simulink model "GammaandTorqueMover"  (R2022b)
settings: Solver=FixedStepAuto  StartTime=0.0  StopTime=10  FixedStep=0.01  RelTol=1e-3
undefined symbols (not defined in the file or in its folder): Kd, Ki, Kp
libraries: mpclib x6, slpidlib x6, simulink x1
(part 2 of 4)

== system GammaandTorqueMover/Tube MPC/MLPM Plant1 ==
  PID Control effort : Inport
  position : Inport  Port=2
  Gamma : Subsystem
  Gravity : Constant  Value=[0;0;-647.2369;0;0;0]
  MATLAB Function : MATLAB Function  TreatAsAtomicUnit=on
  PINV : Subsystem
  Sum1 : Sum  Inputs=++|
  PID Net Wrench : Outport
  PID states : Outport  Port=2
  PID Position and Orientation : Outport  Port=3
  wires:
  Sum1/1 -> MATLAB Function/1(u), PID Net Wrench/1  "PID Net Wrench"
  Gravity/1 -> Sum1/1
  MATLAB Function/2(y) -> PID Position and Orientation/1  "PID Position and Orientation"
  PID Control effort/1 -> PINV/1(input)
  PINV/1(Current) -> Gamma/1(input)  "PID Currents"
  position/1 -> PINV/2(position), Gamma/2(position), MATLAB Function/2(x)
  Gamma/1(net_wrench) -> Sum1/2  "PID Net Wrench"
  MATLAB Function/1(xdot) -> PID states/1  "PID states"

== system GammaandTorqueMover/Tube MPC/Subsystem ==
  Open Loop effort : Inport
  position : Inport  Port=2
  Band-Limited White Noise : simulink/Sources/Band-Limited White Noise  Cov=[0.1]  Ts=0.1  seed=[23341]
  Gamma : Subsystem
  Integrator : Integrator  InitialCondition=[0;0;0;0;0;0;0;0;0;0;0;0]  LimitOutput=on  UpperSaturationLimit=5  LowerSaturationLimit=-5
  MATLAB Function : MATLAB Function  TreatAsAtomicUnit=on
  PINV : Subsystem
  Open Loop Net Wrench : Outport
  Open Loop states : Outport  Port=2
  Open Loop Position and Orientation : Outport  Port=3
  wires:
  Integrator/1 -> Open Loop states/1  "Open Loop states"
  Gamma/1(net_wrench) -> Open Loop Net Wrench/1, MATLAB Function/1(u)  "Open Loop Wrench"
  PINV/1(Current) -> Gamma/1(input)  "Open Loop Currents"
  Open Loop effort/1 -> PINV/1(input)
  MATLAB Function/2(y) -> Open Loop Position and Orientation/1  "Open Loop Position and Orientation"
  position/1 -> MATLAB Function/2(x), Gamma/2(position), PINV/2(position)
  MATLAB Function/1(xdot) -> Integrator/1  "Open Loop states"

== system GammaandTorqueMover/Disturbance added/Linear MPC plus D/MLPM Plant1 ==
  PID Control effort : Inport
  position : Inport  Port=2
  Gamma : Subsystem
  Gravity : Constant  Value=[0;0;-647.2369;0;0;0]
  MATLAB Function : MATLAB Function  TreatAsAtomicUnit=on
  PINV : Subsystem
  Sum1 : Sum  Inputs=++|
  PID Net Wrench : Outport
  PID states : Outport  Port=2
  PID Position and Orientation : Outport  Port=3
  wires:
  Sum1/1 -> MATLAB Function/1(u), PID Net Wrench/1  "PID Net Wrench"
  Gravity/1 -> Sum1/1
  MATLAB Function/2(y) -> PID Position and Orientation/1  "PID Position and Orientation"
  PID Control effort/1 -> PINV/1(input)
  PINV/1(Current) -> Gamma/1(input)  "PID Currents"
  position/1 -> PINV/2(position), Gamma/2(position), MATLAB Function/2(x)
  Gamma/1(net_wrench) -> Sum1/2  "PID Net Wrench"
  MATLAB Function/1(xdot) -> PID states/1  "PID states"

== system GammaandTorqueMover/Disturbance added/Linear MPC plus D/Subsystem ==
  Open Loop effort : Inport
  position : Inport  Port=2
  Gamma : Subsystem
  Integrator : Integrator  InitialCondition=[0;0;0;0;0;0;0;0;0;0;0;0]  LimitOutput=on  UpperSaturationLimit=5  LowerSaturationLimit=-5
  MATLAB Function : MATLAB Function  TreatAsAtomicUnit=on
  Mux2 : Mux  Inputs=6
  PINV : Subsystem
  Step : Step  Time=3  After=1000  SampleTime=0
  Sum : Sum  Inputs=++|
  Open Loop Net Wrench : Outport
  Open Loop states : Outport  Port=2
  Open Loop Position and Orientation : Outport  Port=3
  wires:
  MATLAB Function/1(xdot) -> Integrator/1  "Open Loop states"
  position/1 -> PINV/2(position), Gamma/2(position), MATLAB Function/2(x)
  MATLAB Function/2(y) -> Open Loop Position and Orientation/1  "Open Loop Position and Orientation"
  Open Loop effort/1 -> PINV/1(input)
  PINV/1(Current) -> Gamma/1(input)  "Open Loop Currents"
  Gamma/1(net_wrench) -> Sum/2, Open Loop Net Wrench/1  "Open Loop Wrench"
  Integrator/1 -> Open Loop states/1  "Open Loop states"
  Step/1 -> Mux2/4, Mux2/5, Mux2/6, Mux2/3, Mux2/2, Mux2/1
  Mux2/1 -> Sum/1  "Open loop Disturbance"
  Sum/1 -> MATLAB Function/1(u)

== system GammaandTorqueMover/Disturbance added/PID plus D/MLPM Plant1 ==
  PID Control effort : Inport
  position : Inport  Port=2
  Gamma : Subsystem
  Gravity : Constant  Value=[0;0;-647.2369;0;0;0]
  MATLAB Function : MATLAB Function  TreatAsAtomicUnit=on
  PINV : Subsystem
  Sum1 : Sum  Inputs=++|
  PID Net Wrench : Outport
  PID states : Outport  Port=2
  PID Position and Orientation : Outport  Port=3
  wires:
  MATLAB Function/1(xdot) -> PID states/1  "PID states"
  Gamma/1(net_wrench) -> Sum1/2  "PID Net Wrench"
  position/1 -> MATLAB Function/2(x), Gamma/2(position), PINV/2(position)
  PINV/1(Current) -> Gamma/1(input)  "PID Currents"
  PID Control effort/1 -> PINV/1(input)
  MATLAB Function/2(y) -> PID Position and Orientation/1  "PID Position and Orientation"
  Gravity/1 -> Sum1/1
  Sum1/1 -> PID Net Wrench/1, MATLAB Function/1(u)  "PID Net Wrench"

== system GammaandTorqueMover/Disturbance added/PID plus D/Subsystem ==
  Open Loop effort : Inport
  position : Inport  Port=2
  Gamma : Subsystem
  Integrator : Integrator  InitialCondition=[0;0;0;0;0;0;0;0;0;0;0;0]  LimitOutput=on  UpperSaturationLimit=5  LowerSaturationLimit=-5
  MATLAB Function : MATLAB Function  TreatAsAtomicUnit=on
  Mux2 : Mux  Inputs=6
  PINV : Subsystem
  Step : Step  Time=3  After=1000  SampleTime=0
  Sum : Sum  Inputs=++|
  Open Loop Net Wrench : Outport
  Open Loop states : Outport  Port=2
  Open Loop Position and Orientation : Outport  Port=3
  wires:
  MATLAB Function/1(xdot) -> Integrator/1  "Open Loop states"
  position/1 -> PINV/2(position), Gamma/2(position), MATLAB Function/2(x)
  MATLAB Function/2(y) -> Open Loop Position and Orientation/1  "Open Loop Position and Orientation"
  Open Loop effort/1 -> PINV/1(input)
  PINV/1(Current) -> Gamma/1(input)  "Open Loop Currents"
  Gamma/1(net_wrench) -> Sum/2, Open Loop Net Wrench/1  "Open Loop Wrench"
  Integrator/1 -> Open Loop states/1  "Open Loop states"
  Step/1 -> Mux2/4, Mux2/5, Mux2/6, Mux2/3, Mux2/2, Mux2/1
  Mux2/1 -> Sum/1  "Open loop Disturbance"
  Sum/1 -> MATLAB Function/1(u)

== system GammaandTorqueMover/Disturbance added/Tube MPC plus D/MLPM Plant1 ==
  PID Control effort : Inport
  position : Inport  Port=2
  Gamma : Subsystem
  Gravity : Constant  Value=[0;0;-647.2369;0;0;0]
  MATLAB Function : MATLAB Function  TreatAsAtomicUnit=on
  PINV : Subsystem
  Sum1 : Sum  Inputs=++|
  PID Net Wrench : Outport
  PID states : Outport  Port=2
  PID Position and Orientation : Outport  Port=3
  wires:
  MATLAB Function/1(xdot) -> PID states/1  "PID states"
  Gamma/1(net_wrench) -> Sum1/2  "PID Net Wrench"
  position/1 -> MATLAB Function/2(x), Gamma/2(position), PINV/2(position)
  PINV/1(Current) -> Gamma/1(input)  "PID Currents"
  PID Control effort/1 -> PINV/1(input)
  MATLAB Function/2(y) -> PID Position and Orientation/1  "PID Position and Orientation"
  Gravity/1 -> Sum1/1
  Sum1/1 -> PID Net Wrench/1, MATLAB Function/1(u)  "PID Net Wrench"

== system GammaandTorqueMover/Disturbance added/Tube MPC plus D/Subsystem ==
  Open Loop effort : Inport
  position : Inport  Port=2
  Gamma : Subsystem
  Integrator : Integrator  InitialCondition=[0;0;0;0;0;0;0;0;0;0;0;0]  LimitOutput=on  UpperSaturationLimit=5  LowerSaturationLimit=-5
  MATLAB Function : MATLAB Function  TreatAsAtomicUnit=on
  Mux2 : Mux  Inputs=6
  PINV : Subsystem
  Step : Step  Time=3  After=1000  SampleTime=0
  Sum : Sum  Inputs=++|
  Open Loop Net Wrench : Outport
  Open Loop states : Outport  Port=2
  Open Loop Position and Orientation : Outport  Port=3
  wires:
  MATLAB Function/1(xdot) -> Integrator/1  "Open Loop states"
  position/1 -> PINV/2(position), Gamma/2(position), MATLAB Function/2(x)
  MATLAB Function/2(y) -> Open Loop Position and Orientation/1  "Open Loop Position and Orientation"
  Open Loop effort/1 -> PINV/1(input)
  PINV/1(Current) -> Gamma/1(input)  "Open Loop Currents"
  Gamma/1(net_wrench) -> Sum/2, Open Loop Net Wrench/1  "Open Loop Wrench"
  Integrator/1 -> Open Loop states/1  "Open Loop states"
  Step/1 -> Mux2/4, Mux2/5, Mux2/6, Mux2/3, Mux2/2, Mux2/1
  Mux2/1 -> Sum/1  "Open loop Disturbance"
  Sum/1 -> MATLAB Function/1(u)

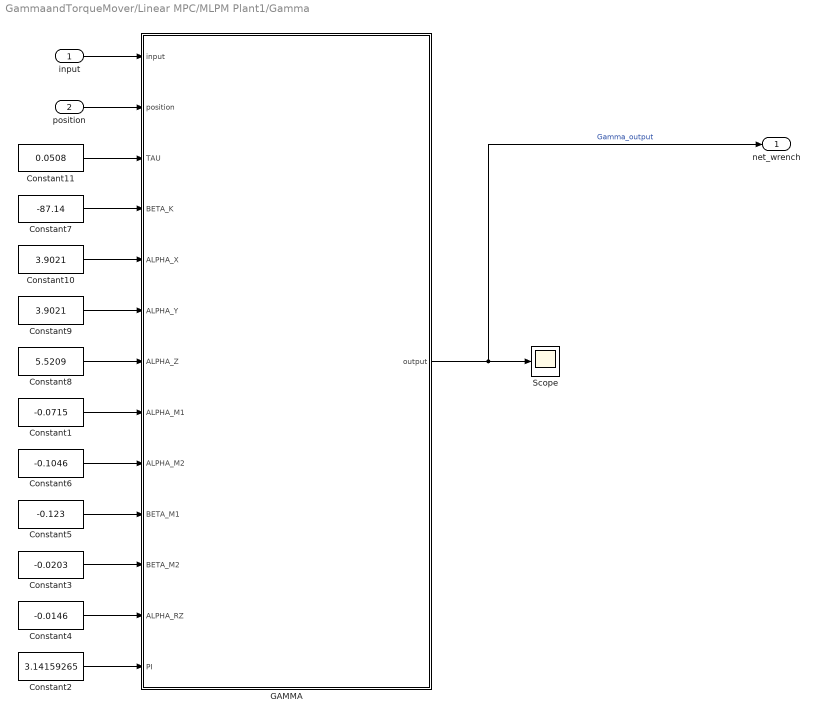
== system GammaandTorqueMover/Linear MPC/MLPM Plant1/Gamma ==
  input : Inport
  position : Inport  Port=2
  Constant1 : Constant  Value=-0.0715
  Constant10 : Constant  Value=3.9021
  Constant11 : Constant  Value=0.0508
  Constant2 : Constant  Value=3.14159265
  Constant3 : Constant  Value=-0.0203
  Constant4 : Constant  Value=-0.0146
  Constant5 : Constant  Value=-0.123
  Constant6 : Constant  Value=-0.1046
  Constant7 : Constant  Value=-87.14
  Constant8 : Constant  Value=5.5209
  Constant9 : Constant  Value=3.9021
  GAMMA : MATLAB Function  TreatAsAtomicUnit=on
  Scope : Scope
  net_wrench : Outport
  wires:
  GAMMA/1(output) -> Scope/1, net_wrench/1  "Gamma_output"
  Constant4/1 -> GAMMA/12(ALPHA_RZ)
  Constant3/1 -> GAMMA/11(BETA_M2)
  Constant5/1 -> GAMMA/10(BETA_M1)
  Constant6/1 -> GAMMA/9(ALPHA_M2)
  Constant1/1 -> GAMMA/8(ALPHA_M1)
  Constant8/1 -> GAMMA/7(ALPHA_Z)
  Constant9/1 -> GAMMA/6(ALPHA_Y)
  Constant10/1 -> GAMMA/5(ALPHA_X)
  Constant7/1 -> GAMMA/4(BETA_K)
  Constant11/1 -> GAMMA/3(TAU)
  Constant2/1 -> GAMMA/13(PI)
  position/1 -> GAMMA/2(position)
  input/1 -> GAMMA/1(input)

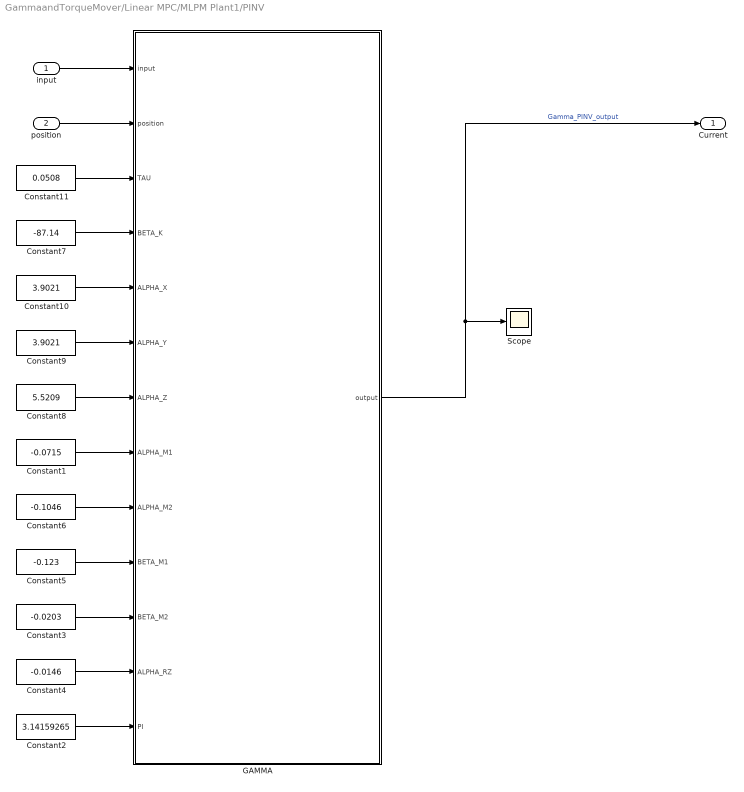
== system GammaandTorqueMover/Linear MPC/MLPM Plant1/PINV ==
  input : Inport
  position : Inport  Port=2
  Constant1 : Constant  Value=-0.0715
  Constant10 : Constant  Value=3.9021
  Constant11 : Constant  Value=0.0508
  Constant2 : Constant  Value=3.14159265
  Constant3 : Constant  Value=-0.0203
  Constant4 : Constant  Value=-0.0146
  Constant5 : Constant  Value=-0.123
  Constant6 : Constant  Value=-0.1046
  Constant7 : Constant  Value=-87.14
  Constant8 : Constant  Value=5.5209
  Constant9 : Constant  Value=3.9021
  GAMMA : MATLAB Function  TreatAsAtomicUnit=on
  Scope : Scope
  Current : Outport
  wires:
  GAMMA/1(output) -> Scope/1, Current/1  "Gamma_PINV_output"
  input/1 -> GAMMA/1(input)
  position/1 -> GAMMA/2(position)
  Constant2/1 -> GAMMA/13(PI)
  Constant11/1 -> GAMMA/3(TAU)
  Constant7/1 -> GAMMA/4(BETA_K)
  Constant10/1 -> GAMMA/5(ALPHA_X)
  Constant9/1 -> GAMMA/6(ALPHA_Y)
  Constant8/1 -> GAMMA/7(ALPHA_Z)
  Constant1/1 -> GAMMA/8(ALPHA_M1)
  Constant6/1 -> GAMMA/9(ALPHA_M2)
  Constant5/1 -> GAMMA/10(BETA_M1)
  Constant3/1 -> GAMMA/11(BETA_M2)
  Constant4/1 -> GAMMA/12(ALPHA_RZ)

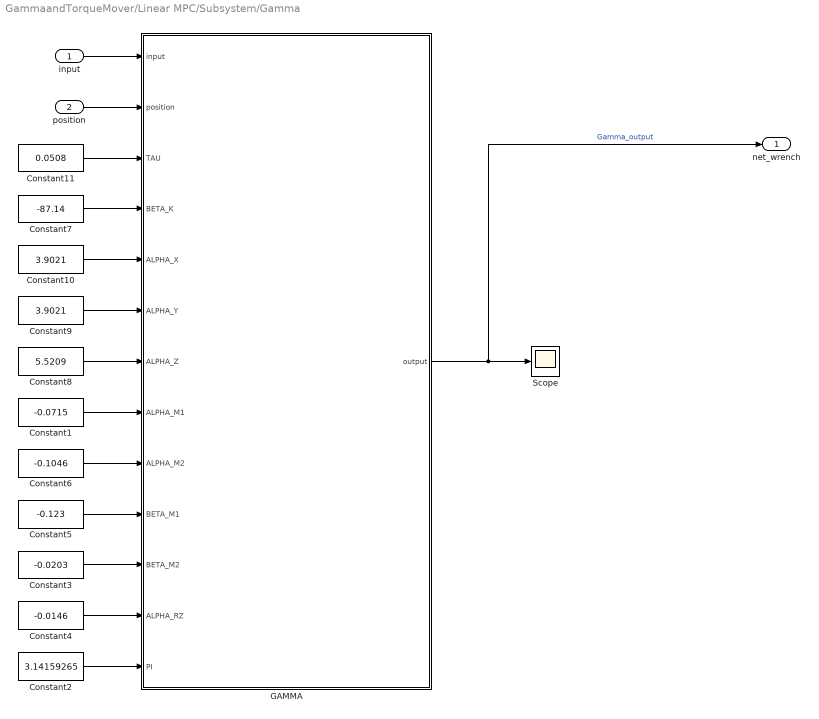
== system GammaandTorqueMover/Linear MPC/Subsystem/Gamma ==
  input : Inport
  position : Inport  Port=2
  Constant1 : Constant  Value=-0.0715
  Constant10 : Constant  Value=3.9021
  Constant11 : Constant  Value=0.0508
  Constant2 : Constant  Value=3.14159265
  Constant3 : Constant  Value=-0.0203
  Constant4 : Constant  Value=-0.0146
  Constant5 : Constant  Value=-0.123
  Constant6 : Constant  Value=-0.1046
  Constant7 : Constant  Value=-87.14
  Constant8 : Constant  Value=5.5209
  Constant9 : Constant  Value=3.9021
  GAMMA : MATLAB Function  TreatAsAtomicUnit=on
  Scope : Scope
  net_wrench : Outport
  wires:
  input/1 -> GAMMA/1(input)
  position/1 -> GAMMA/2(position)
  Constant2/1 -> GAMMA/13(PI)
  Constant11/1 -> GAMMA/3(TAU)
  Constant7/1 -> GAMMA/4(BETA_K)
  Constant10/1 -> GAMMA/5(ALPHA_X)
  Constant9/1 -> GAMMA/6(ALPHA_Y)
  Constant8/1 -> GAMMA/7(ALPHA_Z)
  Constant1/1 -> GAMMA/8(ALPHA_M1)
  Constant6/1 -> GAMMA/9(ALPHA_M2)
  Constant5/1 -> GAMMA/10(BETA_M1)
  Constant3/1 -> GAMMA/11(BETA_M2)
  Constant4/1 -> GAMMA/12(ALPHA_RZ)
  GAMMA/1(output) -> net_wrench/1, Scope/1  "Gamma_output"

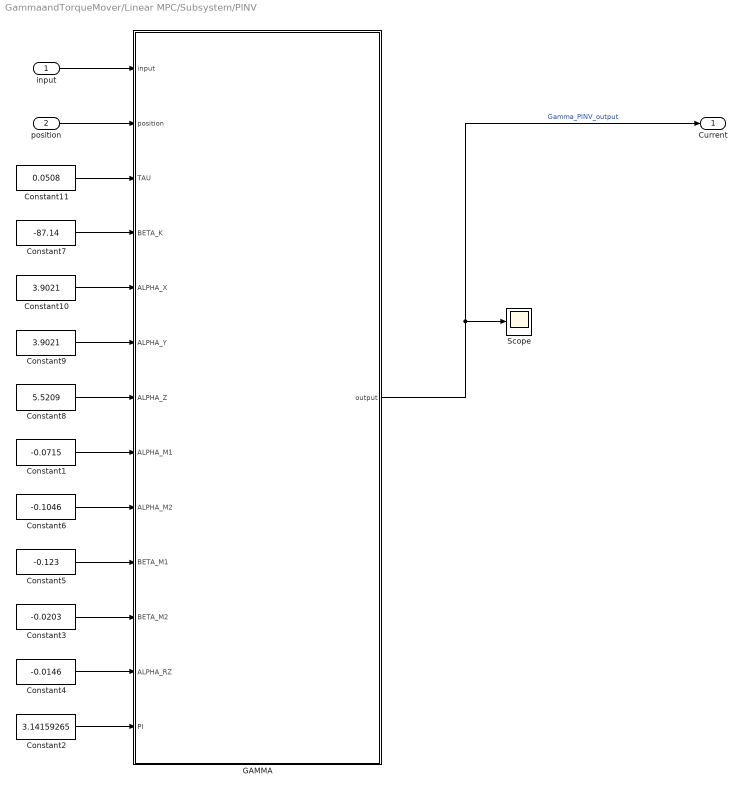
== system GammaandTorqueMover/Linear MPC/Subsystem/PINV ==
  input : Inport
  position : Inport  Port=2
  Constant1 : Constant  Value=-0.0715
  Constant10 : Constant  Value=3.9021
  Constant11 : Constant  Value=0.0508
  Constant2 : Constant  Value=3.14159265
  Constant3 : Constant  Value=-0.0203
  Constant4 : Constant  Value=-0.0146
  Constant5 : Constant  Value=-0.123
  Constant6 : Constant  Value=-0.1046
  Constant7 : Constant  Value=-87.14
  Constant8 : Constant  Value=5.5209
  Constant9 : Constant  Value=3.9021
  GAMMA : MATLAB Function  TreatAsAtomicUnit=on
  Scope : Scope
  Current : Outport
  wires:
  Constant4/1 -> GAMMA/12(ALPHA_RZ)
  Constant3/1 -> GAMMA/11(BETA_M2)
  Constant5/1 -> GAMMA/10(BETA_M1)
  Constant6/1 -> GAMMA/9(ALPHA_M2)
  Constant1/1 -> GAMMA/8(ALPHA_M1)
  Constant8/1 -> GAMMA/7(ALPHA_Z)
  Constant9/1 -> GAMMA/6(ALPHA_Y)
  Constant10/1 -> GAMMA/5(ALPHA_X)
  Constant7/1 -> GAMMA/4(BETA_K)
  Constant11/1 -> GAMMA/3(TAU)
  Constant2/1 -> GAMMA/13(PI)
  position/1 -> GAMMA/2(position)
  input/1 -> GAMMA/1(input)
  GAMMA/1(output) -> Current/1, Scope/1  "Gamma_PINV_output"

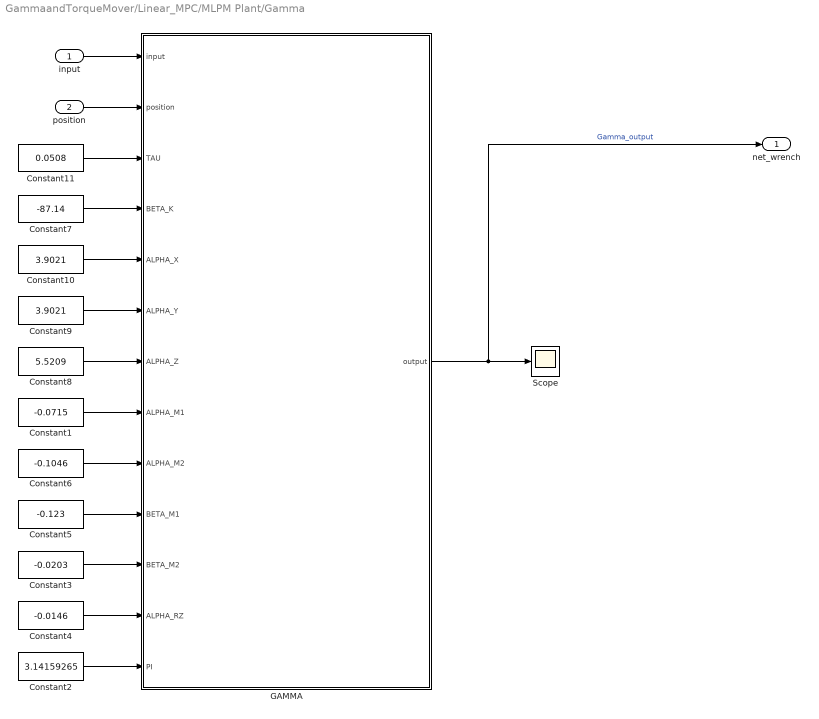
== system GammaandTorqueMover/Linear_MPC/MLPM Plant/Gamma ==
  input : Inport
  position : Inport  Port=2
  Constant1 : Constant  Value=-0.0715
  Constant10 : Constant  Value=3.9021
  Constant11 : Constant  Value=0.0508
  Constant2 : Constant  Value=3.14159265
  Constant3 : Constant  Value=-0.0203
  Constant4 : Constant  Value=-0.0146
  Constant5 : Constant  Value=-0.123
  Constant6 : Constant  Value=-0.1046
  Constant7 : Constant  Value=-87.14
  Constant8 : Constant  Value=5.5209
  Constant9 : Constant  Value=3.9021
  GAMMA : MATLAB Function  TreatAsAtomicUnit=on
  Scope : Scope
  net_wrench : Outport
  wires:
  input/1 -> GAMMA/1(input)
  position/1 -> GAMMA/2(position)
  Constant2/1 -> GAMMA/13(PI)
  Constant11/1 -> GAMMA/3(TAU)
  Constant7/1 -> GAMMA/4(BETA_K)
  Constant10/1 -> GAMMA/5(ALPHA_X)
  Constant9/1 -> GAMMA/6(ALPHA_Y)
  Constant8/1 -> GAMMA/7(ALPHA_Z)
  Constant1/1 -> GAMMA/8(ALPHA_M1)
  Constant6/1 -> GAMMA/9(ALPHA_M2)
  Constant5/1 -> GAMMA/10(BETA_M1)
  Constant3/1 -> GAMMA/11(BETA_M2)
  Constant4/1 -> GAMMA/12(ALPHA_RZ)
  GAMMA/1(output) -> net_wrench/1, Scope/1  "Gamma_output"

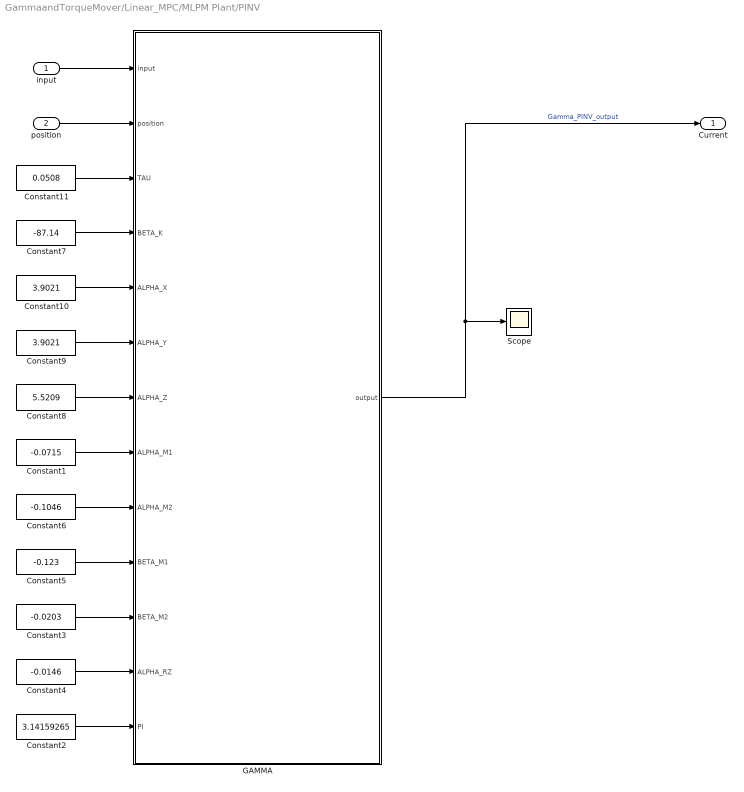
== system GammaandTorqueMover/Linear_MPC/MLPM Plant/PINV ==
  input : Inport
  position : Inport  Port=2
  Constant1 : Constant  Value=-0.0715
  Constant10 : Constant  Value=3.9021
  Constant11 : Constant  Value=0.0508
  Constant2 : Constant  Value=3.14159265
  Constant3 : Constant  Value=-0.0203
  Constant4 : Constant  Value=-0.0146
  Constant5 : Constant  Value=-0.123
  Constant6 : Constant  Value=-0.1046
  Constant7 : Constant  Value=-87.14
  Constant8 : Constant  Value=5.5209
  Constant9 : Constant  Value=3.9021
  GAMMA : MATLAB Function  TreatAsAtomicUnit=on
  Scope : Scope
  Current : Outport
  wires:
  Constant4/1 -> GAMMA/12(ALPHA_RZ)
  Constant3/1 -> GAMMA/11(BETA_M2)
  Constant5/1 -> GAMMA/10(BETA_M1)
  Constant6/1 -> GAMMA/9(ALPHA_M2)
  Constant1/1 -> GAMMA/8(ALPHA_M1)
  Constant8/1 -> GAMMA/7(ALPHA_Z)
  Constant9/1 -> GAMMA/6(ALPHA_Y)
  Constant10/1 -> GAMMA/5(ALPHA_X)
  Constant7/1 -> GAMMA/4(BETA_K)
  Constant11/1 -> GAMMA/3(TAU)
  Constant2/1 -> GAMMA/13(PI)
  position/1 -> GAMMA/2(position)
  input/1 -> GAMMA/1(input)
  GAMMA/1(output) -> Current/1, Scope/1  "Gamma_PINV_output"

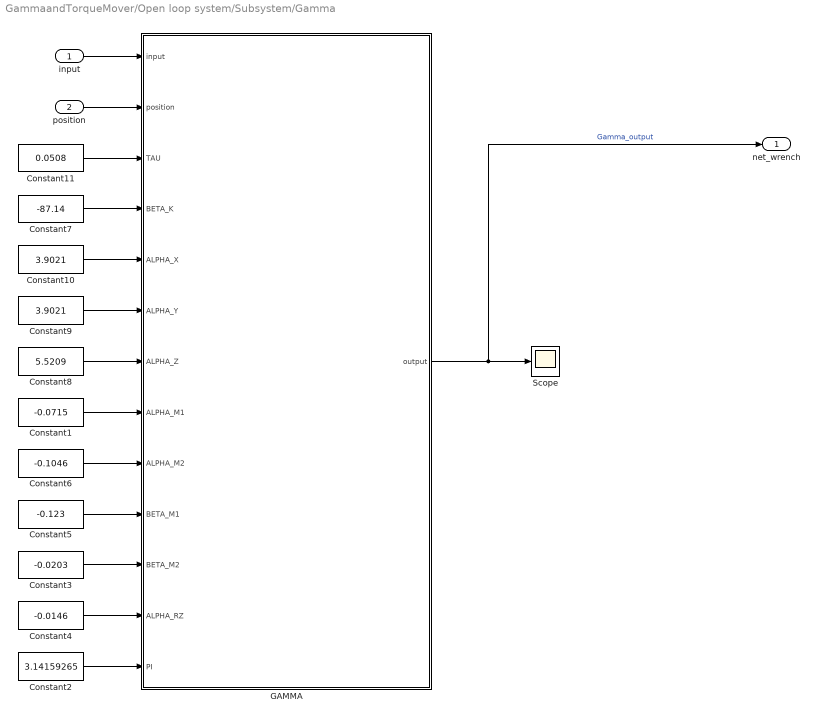
== system GammaandTorqueMover/Open loop system/Subsystem/Gamma ==
  input : Inport
  position : Inport  Port=2
  Constant1 : Constant  Value=-0.0715
  Constant10 : Constant  Value=3.9021
  Constant11 : Constant  Value=0.0508
  Constant2 : Constant  Value=3.14159265
  Constant3 : Constant  Value=-0.0203
  Constant4 : Constant  Value=-0.0146
  Constant5 : Constant  Value=-0.123
  Constant6 : Constant  Value=-0.1046
  Constant7 : Constant  Value=-87.14
  Constant8 : Constant  Value=5.5209
  Constant9 : Constant  Value=3.9021
  GAMMA : MATLAB Function  TreatAsAtomicUnit=on
  Scope : Scope
  net_wrench : Outport
  wires:
  GAMMA/1(output) -> Scope/1, net_wrench/1  "Gamma_output"
  Constant4/1 -> GAMMA/12(ALPHA_RZ)
  Constant3/1 -> GAMMA/11(BETA_M2)
  Constant5/1 -> GAMMA/10(BETA_M1)
  Constant6/1 -> GAMMA/9(ALPHA_M2)
  Constant1/1 -> GAMMA/8(ALPHA_M1)
  Constant8/1 -> GAMMA/7(ALPHA_Z)
  Constant9/1 -> GAMMA/6(ALPHA_Y)
  Constant10/1 -> GAMMA/5(ALPHA_X)
  Constant7/1 -> GAMMA/4(BETA_K)
  Constant11/1 -> GAMMA/3(TAU)
  Constant2/1 -> GAMMA/13(PI)
  position/1 -> GAMMA/2(position)
  input/1 -> GAMMA/1(input)

== system GammaandTorqueMover/Open loop system/Subsystem/PINV ==
  input : Inport
  position : Inport  Port=2
  Constant1 : Constant  Value=-0.0715
  Constant10 : Constant  Value=3.9021
  Constant11 : Constant  Value=0.0508
  Constant2 : Constant  Value=3.14159265
  Constant3 : Constant  Value=-0.0203
  Constant4 : Constant  Value=-0.0146
  Constant5 : Constant  Value=-0.123
  Constant6 : Constant  Value=-0.1046
  Constant7 : Constant  Value=-87.14
  Constant8 : Constant  Value=5.5209
  Constant9 : Constant  Value=3.9021
  GAMMA : MATLAB Function  TreatAsAtomicUnit=on
  Scope : Scope
  Current : Outport
  wires:
  GAMMA/1(output) -> Scope/1, Current/1  "Gamma_PINV_output"
  input/1 -> GAMMA/1(input)
  position/1 -> GAMMA/2(position)
  Constant2/1 -> GAMMA/13(PI)
  Constant11/1 -> GAMMA/3(TAU)
  Constant7/1 -> GAMMA/4(BETA_K)
  Constant10/1 -> GAMMA/5(ALPHA_X)
  Constant9/1 -> GAMMA/6(ALPHA_Y)
  Constant8/1 -> GAMMA/7(ALPHA_Z)
  Constant1/1 -> GAMMA/8(ALPHA_M1)
  Constant6/1 -> GAMMA/9(ALPHA_M2)
  Constant5/1 -> GAMMA/10(BETA_M1)
  Constant3/1 -> GAMMA/11(BETA_M2)
  Constant4/1 -> GAMMA/12(ALPHA_RZ)

== system GammaandTorqueMover/PID/MLPM Plant1/Gamma ==
  input : Inport
  position : Inport  Port=2
  Constant1 : Constant  Value=-0.0715
  Constant10 : Constant  Value=3.9021
  Constant11 : Constant  Value=0.0508
  Constant2 : Constant  Value=3.14159265
  Constant3 : Constant  Value=-0.0203
  Constant4 : Constant  Value=-0.0146
  Constant5 : Constant  Value=-0.123
  Constant6 : Constant  Value=-0.1046
  Constant7 : Constant  Value=-87.14
  Constant8 : Constant  Value=5.5209
  Constant9 : Constant  Value=3.9021
  GAMMA : MATLAB Function  TreatAsAtomicUnit=on
  Scope : Scope
  net_wrench : Outport
  wires:
  input/1 -> GAMMA/1(input)
  position/1 -> GAMMA/2(position)
  Constant2/1 -> GAMMA/13(PI)
  Constant11/1 -> GAMMA/3(TAU)
  Constant7/1 -> GAMMA/4(BETA_K)
  Constant10/1 -> GAMMA/5(ALPHA_X)
  Constant9/1 -> GAMMA/6(ALPHA_Y)
  Constant8/1 -> GAMMA/7(ALPHA_Z)
  Constant1/1 -> GAMMA/8(ALPHA_M1)
  Constant6/1 -> GAMMA/9(ALPHA_M2)
  Constant5/1 -> GAMMA/10(BETA_M1)
  Constant3/1 -> GAMMA/11(BETA_M2)
  Constant4/1 -> GAMMA/12(ALPHA_RZ)
  GAMMA/1(output) -> net_wrench/1, Scope/1  "Gamma_output"

== system GammaandTorqueMover/PID/MLPM Plant1/PINV ==
  input : Inport
  position : Inport  Port=2
  Constant1 : Constant  Value=-0.0715
  Constant10 : Constant  Value=3.9021
  Constant11 : Constant  Value=0.0508
  Constant2 : Constant  Value=3.14159265
  Constant3 : Constant  Value=-0.0203
  Constant4 : Constant  Value=-0.0146
  Constant5 : Constant  Value=-0.123
  Constant6 : Constant  Value=-0.1046
  Constant7 : Constant  Value=-87.14
  Constant8 : Constant  Value=5.5209
  Constant9 : Constant  Value=3.9021
  GAMMA : MATLAB Function  TreatAsAtomicUnit=on
  Scope : Scope
  Current : Outport
  wires:
  Constant4/1 -> GAMMA/12(ALPHA_RZ)
  Constant3/1 -> GAMMA/11(BETA_M2)
  Constant5/1 -> GAMMA/10(BETA_M1)
  Constant6/1 -> GAMMA/9(ALPHA_M2)
  Constant1/1 -> GAMMA/8(ALPHA_M1)
  Constant8/1 -> GAMMA/7(ALPHA_Z)
  Constant9/1 -> GAMMA/6(ALPHA_Y)
  Constant10/1 -> GAMMA/5(ALPHA_X)
  Constant7/1 -> GAMMA/4(BETA_K)
  Constant11/1 -> GAMMA/3(TAU)
  Constant2/1 -> GAMMA/13(PI)
  position/1 -> GAMMA/2(position)
  input/1 -> GAMMA/1(input)
  GAMMA/1(output) -> Current/1, Scope/1  "Gamma_PINV_output"

== system GammaandTorqueMover/PID/Subsystem/Gamma ==
  input : Inport
  position : Inport  Port=2
  Constant1 : Constant  Value=-0.0715
  Constant10 : Constant  Value=3.9021
  Constant11 : Constant  Value=0.0508
  Constant2 : Constant  Value=3.14159265
  Constant3 : Constant  Value=-0.0203
  Constant4 : Constant  Value=-0.0146
  Constant5 : Constant  Value=-0.123
  Constant6 : Constant  Value=-0.1046
  Constant7 : Constant  Value=-87.14
  Constant8 : Constant  Value=5.5209
  Constant9 : Constant  Value=3.9021
  GAMMA : MATLAB Function  TreatAsAtomicUnit=on
  Scope : Scope
  net_wrench : Outport
  wires:
  GAMMA/1(output) -> Scope/1, net_wrench/1  "Gamma_output"
  Constant4/1 -> GAMMA/12(ALPHA_RZ)
  Constant3/1 -> GAMMA/11(BETA_M2)
  Constant5/1 -> GAMMA/10(BETA_M1)
  Constant6/1 -> GAMMA/9(ALPHA_M2)
  Constant1/1 -> GAMMA/8(ALPHA_M1)
  Constant8/1 -> GAMMA/7(ALPHA_Z)
  Constant9/1 -> GAMMA/6(ALPHA_Y)
  Constant10/1 -> GAMMA/5(ALPHA_X)
  Constant7/1 -> GAMMA/4(BETA_K)
  Constant11/1 -> GAMMA/3(TAU)
  Constant2/1 -> GAMMA/13(PI)
  position/1 -> GAMMA/2(position)
  input/1 -> GAMMA/1(input)

== system GammaandTorqueMover/PID/Subsystem/PINV ==
  input : Inport
  position : Inport  Port=2
  Constant1 : Constant  Value=-0.0715
  Constant10 : Constant  Value=3.9021
  Constant11 : Constant  Value=0.0508
  Constant2 : Constant  Value=3.14159265
  Constant3 : Constant  Value=-0.0203
  Constant4 : Constant  Value=-0.0146
  Constant5 : Constant  Value=-0.123
  Constant6 : Constant  Value=-0.1046
  Constant7 : Constant  Value=-87.14
  Constant8 : Constant  Value=5.5209
  Constant9 : Constant  Value=3.9021
  GAMMA : MATLAB Function  TreatAsAtomicUnit=on
  Scope : Scope
  Current : Outport
  wires:
  GAMMA/1(output) -> Scope/1, Current/1  "Gamma_PINV_output"
  input/1 -> GAMMA/1(input)
  position/1 -> GAMMA/2(position)
  Constant2/1 -> GAMMA/13(PI)
  Constant11/1 -> GAMMA/3(TAU)
  Constant7/1 -> GAMMA/4(BETA_K)
  Constant10/1 -> GAMMA/5(ALPHA_X)
  Constant9/1 -> GAMMA/6(ALPHA_Y)
  Constant8/1 -> GAMMA/7(ALPHA_Z)
  Constant1/1 -> GAMMA/8(ALPHA_M1)
  Constant6/1 -> GAMMA/9(ALPHA_M2)
  Constant5/1 -> GAMMA/10(BETA_M1)
  Constant3/1 -> GAMMA/11(BETA_M2)
  Constant4/1 -> GAMMA/12(ALPHA_RZ)

== system GammaandTorqueMover/PID1/MLPM Plant1/Gamma ==
  input : Inport
  position : Inport  Port=2
  Constant1 : Constant  Value=-0.0715
  Constant10 : Constant  Value=3.9021
  Constant11 : Constant  Value=0.0508
  Constant2 : Constant  Value=3.14159265
  Constant3 : Constant  Value=-0.0203
  Constant4 : Constant  Value=-0.0146
  Constant5 : Constant  Value=-0.123
  Constant6 : Constant  Value=-0.1046
  Constant7 : Constant  Value=-87.14
  Constant8 : Constant  Value=5.5209
  Constant9 : Constant  Value=3.9021
  GAMMA : MATLAB Function  TreatAsAtomicUnit=on
  Scope : Scope
  net_wrench : Outport
  wires:
  GAMMA/1(output) -> Scope/1, net_wrench/1  "Gamma_output"
  Constant4/1 -> GAMMA/12(ALPHA_RZ)
  Constant3/1 -> GAMMA/11(BETA_M2)
  Constant5/1 -> GAMMA/10(BETA_M1)
  Constant6/1 -> GAMMA/9(ALPHA_M2)
  Constant1/1 -> GAMMA/8(ALPHA_M1)
  Constant8/1 -> GAMMA/7(ALPHA_Z)
  Constant9/1 -> GAMMA/6(ALPHA_Y)
  Constant10/1 -> GAMMA/5(ALPHA_X)
  Constant7/1 -> GAMMA/4(BETA_K)
  Constant11/1 -> GAMMA/3(TAU)
  Constant2/1 -> GAMMA/13(PI)
  position/1 -> GAMMA/2(position)
  input/1 -> GAMMA/1(input)

== system GammaandTorqueMover/PID1/MLPM Plant1/PINV ==
  input : Inport
  position : Inport  Port=2
  Constant1 : Constant  Value=-0.0715
  Constant10 : Constant  Value=3.9021
  Constant11 : Constant  Value=0.0508
  Constant2 : Constant  Value=3.14159265
  Constant3 : Constant  Value=-0.0203
  Constant4 : Constant  Value=-0.0146
  Constant5 : Constant  Value=-0.123
  Constant6 : Constant  Value=-0.1046
  Constant7 : Constant  Value=-87.14
  Constant8 : Constant  Value=5.5209
  Constant9 : Constant  Value=3.9021
  GAMMA : MATLAB Function  TreatAsAtomicUnit=on
  Scope : Scope
  Current : Outport
  wires:
  GAMMA/1(output) -> Scope/1, Current/1  "Gamma_PINV_output"
  input/1 -> GAMMA/1(input)
  position/1 -> GAMMA/2(position)
  Constant2/1 -> GAMMA/13(PI)
  Constant11/1 -> GAMMA/3(TAU)
  Constant7/1 -> GAMMA/4(BETA_K)
  Constant10/1 -> GAMMA/5(ALPHA_X)
  Constant9/1 -> GAMMA/6(ALPHA_Y)
  Constant8/1 -> GAMMA/7(ALPHA_Z)
  Constant1/1 -> GAMMA/8(ALPHA_M1)
  Constant6/1 -> GAMMA/9(ALPHA_M2)
  Constant5/1 -> GAMMA/10(BETA_M1)
  Constant3/1 -> GAMMA/11(BETA_M2)
  Constant4/1 -> GAMMA/12(ALPHA_RZ)

== system GammaandTorqueMover/PID1/Subsystem/Gamma ==
  input : Inport
  position : Inport  Port=2
  Constant1 : Constant  Value=-0.0715
  Constant10 : Constant  Value=3.9021
  Constant11 : Constant  Value=0.0508
  Constant2 : Constant  Value=3.14159265
  Constant3 : Constant  Value=-0.0203
  Constant4 : Constant  Value=-0.0146
  Constant5 : Constant  Value=-0.123
  Constant6 : Constant  Value=-0.1046
  Constant7 : Constant  Value=-87.14
  Constant8 : Constant  Value=5.5209
  Constant9 : Constant  Value=3.9021
  GAMMA : MATLAB Function  TreatAsAtomicUnit=on
  Scope : Scope
  net_wrench : Outport
  wires:
  input/1 -> GAMMA/1(input)
  position/1 -> GAMMA/2(position)
  Constant2/1 -> GAMMA/13(PI)
  Constant11/1 -> GAMMA/3(TAU)
  Constant7/1 -> GAMMA/4(BETA_K)
  Constant10/1 -> GAMMA/5(ALPHA_X)
  Constant9/1 -> GAMMA/6(ALPHA_Y)
  Constant8/1 -> GAMMA/7(ALPHA_Z)
  Constant1/1 -> GAMMA/8(ALPHA_M1)
  Constant6/1 -> GAMMA/9(ALPHA_M2)
  Constant5/1 -> GAMMA/10(BETA_M1)
  Constant3/1 -> GAMMA/11(BETA_M2)
  Constant4/1 -> GAMMA/12(ALPHA_RZ)
  GAMMA/1(output) -> net_wrench/1, Scope/1  "Gamma_output"

== system GammaandTorqueMover/PID1/Subsystem/PINV ==
  input : Inport
  position : Inport  Port=2
  Constant1 : Constant  Value=-0.0715
  Constant10 : Constant  Value=3.9021
  Constant11 : Constant  Value=0.0508
  Constant2 : Constant  Value=3.14159265
  Constant3 : Constant  Value=-0.0203
  Constant4 : Constant  Value=-0.0146
  Constant5 : Constant  Value=-0.123
  Constant6 : Constant  Value=-0.1046
  Constant7 : Constant  Value=-87.14
  Constant8 : Constant  Value=5.5209
  Constant9 : Constant  Value=3.9021
  GAMMA : MATLAB Function  TreatAsAtomicUnit=on
  Scope : Scope
  Current : Outport
  wires:
  Constant4/1 -> GAMMA/12(ALPHA_RZ)
  Constant3/1 -> GAMMA/11(BETA_M2)
  Constant5/1 -> GAMMA/10(BETA_M1)
  Constant6/1 -> GAMMA/9(ALPHA_M2)
  Constant1/1 -> GAMMA/8(ALPHA_M1)
  Constant8/1 -> GAMMA/7(ALPHA_Z)
  Constant9/1 -> GAMMA/6(ALPHA_Y)
  Constant10/1 -> GAMMA/5(ALPHA_X)
  Constant7/1 -> GAMMA/4(BETA_K)
  Constant11/1 -> GAMMA/3(TAU)
  Constant2/1 -> GAMMA/13(PI)
  position/1 -> GAMMA/2(position)
  input/1 -> GAMMA/1(input)
  GAMMA/1(output) -> Current/1, Scope/1  "Gamma_PINV_output"

== system GammaandTorqueMover/PID2/Subsystem/Gamma ==
  input : Inport
  position : Inport  Port=2
  Constant1 : Constant  Value=-0.0715
  Constant10 : Constant  Value=3.9021
  Constant11 : Constant  Value=0.0508
  Constant2 : Constant  Value=3.14159265
  Constant3 : Constant  Value=-0.0203
  Constant4 : Constant  Value=-0.0146
  Constant5 : Constant  Value=-0.123
  Constant6 : Constant  Value=-0.1046
  Constant7 : Constant  Value=-87.14
  Constant8 : Constant  Value=5.5209
  Constant9 : Constant  Value=3.9021
  GAMMA : MATLAB Function  TreatAsAtomicUnit=on
  Scope : Scope
  net_wrench : Outport
  wires:
  input/1 -> GAMMA/1(input)
  position/1 -> GAMMA/2(position)
  Constant2/1 -> GAMMA/13(PI)
  Constant11/1 -> GAMMA/3(TAU)
  Constant7/1 -> GAMMA/4(BETA_K)
  Constant10/1 -> GAMMA/5(ALPHA_X)
  Constant9/1 -> GAMMA/6(ALPHA_Y)
  Constant8/1 -> GAMMA/7(ALPHA_Z)
  Constant1/1 -> GAMMA/8(ALPHA_M1)
  Constant6/1 -> GAMMA/9(ALPHA_M2)
  Constant5/1 -> GAMMA/10(BETA_M1)
  Constant3/1 -> GAMMA/11(BETA_M2)
  Constant4/1 -> GAMMA/12(ALPHA_RZ)
  GAMMA/1(output) -> net_wrench/1, Scope/1  "Gamma_output"

== system GammaandTorqueMover/PID2/Subsystem/PINV ==
  input : Inport
  position : Inport  Port=2
  Constant1 : Constant  Value=-0.0715
  Constant10 : Constant  Value=3.9021
  Constant11 : Constant  Value=0.0508
  Constant2 : Constant  Value=3.14159265
  Constant3 : Constant  Value=-0.0203
  Constant4 : Constant  Value=-0.0146
  Constant5 : Constant  Value=-0.123
  Constant6 : Constant  Value=-0.1046
  Constant7 : Constant  Value=-87.14
  Constant8 : Constant  Value=5.5209
  Constant9 : Constant  Value=3.9021
  GAMMA : MATLAB Function  TreatAsAtomicUnit=on
  Scope : Scope
  Current : Outport
  wires:
  Constant4/1 -> GAMMA/12(ALPHA_RZ)
  Constant3/1 -> GAMMA/11(BETA_M2)
  Constant5/1 -> GAMMA/10(BETA_M1)
  Constant6/1 -> GAMMA/9(ALPHA_M2)
  Constant1/1 -> GAMMA/8(ALPHA_M1)
  Constant8/1 -> GAMMA/7(ALPHA_Z)
  Constant9/1 -> GAMMA/6(ALPHA_Y)
  Constant10/1 -> GAMMA/5(ALPHA_X)
  Constant7/1 -> GAMMA/4(BETA_K)
  Constant11/1 -> GAMMA/3(TAU)
  Constant2/1 -> GAMMA/13(PI)
  position/1 -> GAMMA/2(position)
  input/1 -> GAMMA/1(input)
  GAMMA/1(output) -> Current/1, Scope/1  "Gamma_PINV_output"

== system GammaandTorqueMover/Tube MPC/MLPM Plant1/Gamma ==
  input : Inport
  position : Inport  Port=2
  Constant1 : Constant  Value=-0.0715
  Constant10 : Constant  Value=3.9021
  Constant11 : Constant  Value=0.0508
  Constant2 : Constant  Value=3.14159265
  Constant3 : Constant  Value=-0.0203
  Constant4 : Constant  Value=-0.0146
  Constant5 : Constant  Value=-0.123
  Constant6 : Constant  Value=-0.1046
  Constant7 : Constant  Value=-87.14
  Constant8 : Constant  Value=5.5209
  Constant9 : Constant  Value=3.9021
  GAMMA : MATLAB Function  TreatAsAtomicUnit=on
  Scope : Scope
  net_wrench : Outport
  wires:
  input/1 -> GAMMA/1(input)
  position/1 -> GAMMA/2(position)
  Constant2/1 -> GAMMA/13(PI)
  Constant11/1 -> GAMMA/3(TAU)
  Constant7/1 -> GAMMA/4(BETA_K)
  Constant10/1 -> GAMMA/5(ALPHA_X)
  Constant9/1 -> GAMMA/6(ALPHA_Y)
  Constant8/1 -> GAMMA/7(ALPHA_Z)
  Constant1/1 -> GAMMA/8(ALPHA_M1)
  Constant6/1 -> GAMMA/9(ALPHA_M2)
  Constant5/1 -> GAMMA/10(BETA_M1)
  Constant3/1 -> GAMMA/11(BETA_M2)
  Constant4/1 -> GAMMA/12(ALPHA_RZ)
  GAMMA/1(output) -> net_wrench/1, Scope/1  "Gamma_output"

== system GammaandTorqueMover/Tube MPC/MLPM Plant1/PINV ==
  input : Inport
  position : Inport  Port=2
  Constant1 : Constant  Value=-0.0715
  Constant10 : Constant  Value=3.9021
  Constant11 : Constant  Value=0.0508
  Constant2 : Constant  Value=3.14159265
  Constant3 : Constant  Value=-0.0203
  Constant4 : Constant  Value=-0.0146
  Constant5 : Constant  Value=-0.123
  Constant6 : Constant  Value=-0.1046
  Constant7 : Constant  Value=-87.14
  Constant8 : Constant  Value=5.5209
  Constant9 : Constant  Value=3.9021
  GAMMA : MATLAB Function  TreatAsAtomicUnit=on
  Scope : Scope
  Current : Outport
  wires:
  Constant4/1 -> GAMMA/12(ALPHA_RZ)
  Constant3/1 -> GAMMA/11(BETA_M2)
  Constant5/1 -> GAMMA/10(BETA_M1)
  Constant6/1 -> GAMMA/9(ALPHA_M2)
  Constant1/1 -> GAMMA/8(ALPHA_M1)
  Constant8/1 -> GAMMA/7(ALPHA_Z)
  Constant9/1 -> GAMMA/6(ALPHA_Y)
  Constant10/1 -> GAMMA/5(ALPHA_X)
  Constant7/1 -> GAMMA/4(BETA_K)
  Constant11/1 -> GAMMA/3(TAU)
  Constant2/1 -> GAMMA/13(PI)
  position/1 -> GAMMA/2(position)
  input/1 -> GAMMA/1(input)
  GAMMA/1(output) -> Current/1, Scope/1  "Gamma_PINV_output"

== system GammaandTorqueMover/Tube MPC/Subsystem/Gamma ==
  input : Inport
  position : Inport  Port=2
  Constant1 : Constant  Value=-0.0715
  Constant10 : Constant  Value=3.9021
  Constant11 : Constant  Value=0.0508
  Constant2 : Constant  Value=3.14159265
  Constant3 : Constant  Value=-0.0203
  Constant4 : Constant  Value=-0.0146
  Constant5 : Constant  Value=-0.123
  Constant6 : Constant  Value=-0.1046
  Constant7 : Constant  Value=-87.14
  Constant8 : Constant  Value=5.5209
  Constant9 : Constant  Value=3.9021
  GAMMA : MATLAB Function  TreatAsAtomicUnit=on
  Scope : Scope
  net_wrench : Outport
  wires:
  GAMMA/1(output) -> Scope/1, net_wrench/1  "Gamma_output"
  Constant4/1 -> GAMMA/12(ALPHA_RZ)
  Constant3/1 -> GAMMA/11(BETA_M2)
  Constant5/1 -> GAMMA/10(BETA_M1)
  Constant6/1 -> GAMMA/9(ALPHA_M2)
  Constant1/1 -> GAMMA/8(ALPHA_M1)
  Constant8/1 -> GAMMA/7(ALPHA_Z)
  Constant9/1 -> GAMMA/6(ALPHA_Y)
  Constant10/1 -> GAMMA/5(ALPHA_X)
  Constant7/1 -> GAMMA/4(BETA_K)
  Constant11/1 -> GAMMA/3(TAU)
  Constant2/1 -> GAMMA/13(PI)
  position/1 -> GAMMA/2(position)
  input/1 -> GAMMA/1(input)

== system GammaandTorqueMover/Tube MPC/Subsystem/PINV ==
  input : Inport
  position : Inport  Port=2
  Constant1 : Constant  Value=-0.0715
  Constant10 : Constant  Value=3.9021
  Constant11 : Constant  Value=0.0508
  Constant2 : Constant  Value=3.14159265
  Constant3 : Constant  Value=-0.0203
  Constant4 : Constant  Value=-0.0146
  Constant5 : Constant  Value=-0.123
  Constant6 : Constant  Value=-0.1046
  Constant7 : Constant  Value=-87.14
  Constant8 : Constant  Value=5.5209
  Constant9 : Constant  Value=3.9021
  GAMMA : MATLAB Function  TreatAsAtomicUnit=on
  Scope : Scope
  Current : Outport
  wires:
  GAMMA/1(output) -> Scope/1, Current/1  "Gamma_PINV_output"
  input/1 -> GAMMA/1(input)
  position/1 -> GAMMA/2(position)
  Constant2/1 -> GAMMA/13(PI)
  Constant11/1 -> GAMMA/3(TAU)
  Constant7/1 -> GAMMA/4(BETA_K)
  Constant10/1 -> GAMMA/5(ALPHA_X)
  Constant9/1 -> GAMMA/6(ALPHA_Y)
  Constant8/1 -> GAMMA/7(ALPHA_Z)
  Constant1/1 -> GAMMA/8(ALPHA_M1)
  Constant6/1 -> GAMMA/9(ALPHA_M2)
  Constant5/1 -> GAMMA/10(BETA_M1)
  Constant3/1 -> GAMMA/11(BETA_M2)
  Constant4/1 -> GAMMA/12(ALPHA_RZ)

== system GammaandTorqueMover/Disturbance added/Linear MPC plus D/MLPM Plant1/Gamma ==
  input : Inport
  position : Inport  Port=2
  Constant1 : Constant  Value=-0.0715
  Constant10 : Constant  Value=3.9021
  Constant11 : Constant  Value=0.0508
  Constant2 : Constant  Value=3.14159265
  Constant3 : Constant  Value=-0.0203
  Constant4 : Constant  Value=-0.0146
  Constant5 : Constant  Value=-0.123
  Constant6 : Constant  Value=-0.1046
  Constant7 : Constant  Value=-87.14
  Constant8 : Constant  Value=5.5209
  Constant9 : Constant  Value=3.9021
  GAMMA : MATLAB Function  TreatAsAtomicUnit=on
  Scope : Scope
  net_wrench : Outport
  wires:
  input/1 -> GAMMA/1(input)
  position/1 -> GAMMA/2(position)
  Constant2/1 -> GAMMA/13(PI)
  Constant11/1 -> GAMMA/3(TAU)
  Constant7/1 -> GAMMA/4(BETA_K)
  Constant10/1 -> GAMMA/5(ALPHA_X)
  Constant9/1 -> GAMMA/6(ALPHA_Y)
  Constant8/1 -> GAMMA/7(ALPHA_Z)
  Constant1/1 -> GAMMA/8(ALPHA_M1)
  Constant6/1 -> GAMMA/9(ALPHA_M2)
  Constant5/1 -> GAMMA/10(BETA_M1)
  Constant3/1 -> GAMMA/11(BETA_M2)
  Constant4/1 -> GAMMA/12(ALPHA_RZ)
  GAMMA/1(output) -> net_wrench/1, Scope/1  "Gamma_output"

== system GammaandTorqueMover/Disturbance added/Linear MPC plus D/MLPM Plant1/PINV ==
  input : Inport
  position : Inport  Port=2
  Constant1 : Constant  Value=-0.0715
  Constant10 : Constant  Value=3.9021
  Constant11 : Constant  Value=0.0508
  Constant2 : Constant  Value=3.14159265
  Constant3 : Constant  Value=-0.0203
  Constant4 : Constant  Value=-0.0146
  Constant5 : Constant  Value=-0.123
  Constant6 : Constant  Value=-0.1046
  Constant7 : Constant  Value=-87.14
  Constant8 : Constant  Value=5.5209
  Constant9 : Constant  Value=3.9021
  GAMMA : MATLAB Function  TreatAsAtomicUnit=on
  Scope : Scope
  Current : Outport
  wires:
  Constant4/1 -> GAMMA/12(ALPHA_RZ)
  Constant3/1 -> GAMMA/11(BETA_M2)
  Constant5/1 -> GAMMA/10(BETA_M1)
  Constant6/1 -> GAMMA/9(ALPHA_M2)
  Constant1/1 -> GAMMA/8(ALPHA_M1)
  Constant8/1 -> GAMMA/7(ALPHA_Z)
  Constant9/1 -> GAMMA/6(ALPHA_Y)
  Constant10/1 -> GAMMA/5(ALPHA_X)
  Constant7/1 -> GAMMA/4(BETA_K)
  Constant11/1 -> GAMMA/3(TAU)
  Constant2/1 -> GAMMA/13(PI)
  position/1 -> GAMMA/2(position)
  input/1 -> GAMMA/1(input)
  GAMMA/1(output) -> Current/1, Scope/1  "Gamma_PINV_output"

== system GammaandTorqueMover/Disturbance added/Linear MPC plus D/Subsystem/Gamma ==
  input : Inport
  position : Inport  Port=2
  Constant1 : Constant  Value=-0.0715
  Constant10 : Constant  Value=3.9021
  Constant11 : Constant  Value=0.0508
  Constant2 : Constant  Value=3.14159265
  Constant3 : Constant  Value=-0.0203
  Constant4 : Constant  Value=-0.0146
  Constant5 : Constant  Value=-0.123
  Constant6 : Constant  Value=-0.1046
  Constant7 : Constant  Value=-87.14
  Constant8 : Constant  Value=5.5209
  Constant9 : Constant  Value=3.9021
  GAMMA : MATLAB Function  TreatAsAtomicUnit=on
  Scope : Scope
  net_wrench : Outport
  wires:
  input/1 -> GAMMA/1(input)
  position/1 -> GAMMA/2(position)
  Constant2/1 -> GAMMA/13(PI)
  Constant11/1 -> GAMMA/3(TAU)
  Constant7/1 -> GAMMA/4(BETA_K)
  Constant10/1 -> GAMMA/5(ALPHA_X)
  Constant9/1 -> GAMMA/6(ALPHA_Y)
  Constant8/1 -> GAMMA/7(ALPHA_Z)
  Constant1/1 -> GAMMA/8(ALPHA_M1)
  Constant6/1 -> GAMMA/9(ALPHA_M2)
  Constant5/1 -> GAMMA/10(BETA_M1)
  Constant3/1 -> GAMMA/11(BETA_M2)
  Constant4/1 -> GAMMA/12(ALPHA_RZ)
  GAMMA/1(output) -> net_wrench/1, Scope/1  "Gamma_output"

== system GammaandTorqueMover/Disturbance added/Linear MPC plus D/Subsystem/PINV ==
  input : Inport
  position : Inport  Port=2
  Constant1 : Constant  Value=-0.0715
  Constant10 : Constant  Value=3.9021
  Constant11 : Constant  Value=0.0508
  Constant2 : Constant  Value=3.14159265
  Constant3 : Constant  Value=-0.0203
  Constant4 : Constant  Value=-0.0146
  Constant5 : Constant  Value=-0.123
  Constant6 : Constant  Value=-0.1046
  Constant7 : Constant  Value=-87.14
  Constant8 : Constant  Value=5.5209
  Constant9 : Constant  Value=3.9021
  GAMMA : MATLAB Function  TreatAsAtomicUnit=on
  Scope : Scope
  Current : Outport
  wires:
  Constant4/1 -> GAMMA/12(ALPHA_RZ)
  Constant3/1 -> GAMMA/11(BETA_M2)
  Constant5/1 -> GAMMA/10(BETA_M1)
  Constant6/1 -> GAMMA/9(ALPHA_M2)
  Constant1/1 -> GAMMA/8(ALPHA_M1)
  Constant8/1 -> GAMMA/7(ALPHA_Z)
  Constant9/1 -> GAMMA/6(ALPHA_Y)
  Constant10/1 -> GAMMA/5(ALPHA_X)
  Constant7/1 -> GAMMA/4(BETA_K)
  Constant11/1 -> GAMMA/3(TAU)
  Constant2/1 -> GAMMA/13(PI)
  position/1 -> GAMMA/2(position)
  input/1 -> GAMMA/1(input)
  GAMMA/1(output) -> Current/1, Scope/1  "Gamma_PINV_output"

== system GammaandTorqueMover/Disturbance added/PID plus D/MLPM Plant1/Gamma ==
  input : Inport
  position : Inport  Port=2
  Constant1 : Constant  Value=-0.0715
  Constant10 : Constant  Value=3.9021
  Constant11 : Constant  Value=0.0508
  Constant2 : Constant  Value=3.14159265
  Constant3 : Constant  Value=-0.0203
  Constant4 : Constant  Value=-0.0146
  Constant5 : Constant  Value=-0.123
  Constant6 : Constant  Value=-0.1046
  Constant7 : Constant  Value=-87.14
  Constant8 : Constant  Value=5.5209
  Constant9 : Constant  Value=3.9021
  GAMMA : MATLAB Function  TreatAsAtomicUnit=on
  Scope : Scope
  net_wrench : Outport
  wires:
  GAMMA/1(output) -> Scope/1, net_wrench/1  "Gamma_output"
  Constant4/1 -> GAMMA/12(ALPHA_RZ)
  Constant3/1 -> GAMMA/11(BETA_M2)
  Constant5/1 -> GAMMA/10(BETA_M1)
  Constant6/1 -> GAMMA/9(ALPHA_M2)
  Constant1/1 -> GAMMA/8(ALPHA_M1)
  Constant8/1 -> GAMMA/7(ALPHA_Z)
  Constant9/1 -> GAMMA/6(ALPHA_Y)
  Constant10/1 -> GAMMA/5(ALPHA_X)
  Constant7/1 -> GAMMA/4(BETA_K)
  Constant11/1 -> GAMMA/3(TAU)
  Constant2/1 -> GAMMA/13(PI)
  position/1 -> GAMMA/2(position)
  input/1 -> GAMMA/1(input)

== system GammaandTorqueMover/Disturbance added/PID plus D/MLPM Plant1/PINV ==
  input : Inport
  position : Inport  Port=2
  Constant1 : Constant  Value=-0.0715
  Constant10 : Constant  Value=3.9021
  Constant11 : Constant  Value=0.0508
  Constant2 : Constant  Value=3.14159265
  Constant3 : Constant  Value=-0.0203
  Constant4 : Constant  Value=-0.0146
  Constant5 : Constant  Value=-0.123
  Constant6 : Constant  Value=-0.1046
  Constant7 : Constant  Value=-87.14
  Constant8 : Constant  Value=5.5209
  Constant9 : Constant  Value=3.9021
  GAMMA : MATLAB Function  TreatAsAtomicUnit=on
  Scope : Scope
  Current : Outport
  wires:
  GAMMA/1(output) -> Scope/1, Current/1  "Gamma_PINV_output"
  input/1 -> GAMMA/1(input)
  position/1 -> GAMMA/2(position)
  Constant2/1 -> GAMMA/13(PI)
  Constant11/1 -> GAMMA/3(TAU)
  Constant7/1 -> GAMMA/4(BETA_K)
  Constant10/1 -> GAMMA/5(ALPHA_X)
  Constant9/1 -> GAMMA/6(ALPHA_Y)
  Constant8/1 -> GAMMA/7(ALPHA_Z)
  Constant1/1 -> GAMMA/8(ALPHA_M1)
  Constant6/1 -> GAMMA/9(ALPHA_M2)
  Constant5/1 -> GAMMA/10(BETA_M1)
  Constant3/1 -> GAMMA/11(BETA_M2)
  Constant4/1 -> GAMMA/12(ALPHA_RZ)

== system GammaandTorqueMover/Disturbance added/PID plus D/Subsystem/Gamma ==
  input : Inport
  position : Inport  Port=2
  Constant1 : Constant  Value=-0.0715
  Constant10 : Constant  Value=3.9021
  Constant11 : Constant  Value=0.0508
  Constant2 : Constant  Value=3.14159265
  Constant3 : Constant  Value=-0.0203
  Constant4 : Constant  Value=-0.0146
  Constant5 : Constant  Value=-0.123
  Constant6 : Constant  Value=-0.1046
  Constant7 : Constant  Value=-87.14
  Constant8 : Constant  Value=5.5209
  Constant9 : Constant  Value=3.9021
  GAMMA : MATLAB Function  TreatAsAtomicUnit=on
  Scope : Scope
  net_wrench : Outport
  wires:
  input/1 -> GAMMA/1(input)
  position/1 -> GAMMA/2(position)
  Constant2/1 -> GAMMA/13(PI)
  Constant11/1 -> GAMMA/3(TAU)
  Constant7/1 -> GAMMA/4(BETA_K)
  Constant10/1 -> GAMMA/5(ALPHA_X)
  Constant9/1 -> GAMMA/6(ALPHA_Y)
  Constant8/1 -> GAMMA/7(ALPHA_Z)
  Constant1/1 -> GAMMA/8(ALPHA_M1)
  Constant6/1 -> GAMMA/9(ALPHA_M2)
  Constant5/1 -> GAMMA/10(BETA_M1)
  Constant3/1 -> GAMMA/11(BETA_M2)
  Constant4/1 -> GAMMA/12(ALPHA_RZ)
  GAMMA/1(output) -> net_wrench/1, Scope/1  "Gamma_output"

== system GammaandTorqueMover/Disturbance added/PID plus D/Subsystem/PINV ==
  input : Inport
  position : Inport  Port=2
  Constant1 : Constant  Value=-0.0715
  Constant10 : Constant  Value=3.9021
  Constant11 : Constant  Value=0.0508
  Constant2 : Constant  Value=3.14159265
  Constant3 : Constant  Value=-0.0203
  Constant4 : Constant  Value=-0.0146
  Constant5 : Constant  Value=-0.123
  Constant6 : Constant  Value=-0.1046
  Constant7 : Constant  Value=-87.14
  Constant8 : Constant  Value=5.5209
  Constant9 : Constant  Value=3.9021
  GAMMA : MATLAB Function  TreatAsAtomicUnit=on
  Scope : Scope
  Current : Outport
  wires:
  Constant4/1 -> GAMMA/12(ALPHA_RZ)
  Constant3/1 -> GAMMA/11(BETA_M2)
  Constant5/1 -> GAMMA/10(BETA_M1)
  Constant6/1 -> GAMMA/9(ALPHA_M2)
  Constant1/1 -> GAMMA/8(ALPHA_M1)
  Constant8/1 -> GAMMA/7(ALPHA_Z)
  Constant9/1 -> GAMMA/6(ALPHA_Y)
  Constant10/1 -> GAMMA/5(ALPHA_X)
  Constant7/1 -> GAMMA/4(BETA_K)
  Constant11/1 -> GAMMA/3(TAU)
  Constant2/1 -> GAMMA/13(PI)
  position/1 -> GAMMA/2(position)
  input/1 -> GAMMA/1(input)
  GAMMA/1(output) -> Current/1, Scope/1  "Gamma_PINV_output"

== system GammaandTorqueMover/Disturbance added/Tube MPC plus D/MLPM Plant1/Gamma ==
  input : Inport
  position : Inport  Port=2
  Constant1 : Constant  Value=-0.0715
  Constant10 : Constant  Value=3.9021
  Constant11 : Constant  Value=0.0508
  Constant2 : Constant  Value=3.14159265
  Constant3 : Constant  Value=-0.0203
  Constant4 : Constant  Value=-0.0146
  Constant5 : Constant  Value=-0.123
  Constant6 : Constant  Value=-0.1046
  Constant7 : Constant  Value=-87.14
  Constant8 : Constant  Value=5.5209
  Constant9 : Constant  Value=3.9021
  GAMMA : MATLAB Function  TreatAsAtomicUnit=on
  Scope : Scope
  net_wrench : Outport
  wires:
  GAMMA/1(output) -> Scope/1, net_wrench/1  "Gamma_output"
  Constant4/1 -> GAMMA/12(ALPHA_RZ)
  Constant3/1 -> GAMMA/11(BETA_M2)
  Constant5/1 -> GAMMA/10(BETA_M1)
  Constant6/1 -> GAMMA/9(ALPHA_M2)
  Constant1/1 -> GAMMA/8(ALPHA_M1)
  Constant8/1 -> GAMMA/7(ALPHA_Z)
  Constant9/1 -> GAMMA/6(ALPHA_Y)
  Constant10/1 -> GAMMA/5(ALPHA_X)
  Constant7/1 -> GAMMA/4(BETA_K)
  Constant11/1 -> GAMMA/3(TAU)
  Constant2/1 -> GAMMA/13(PI)
  position/1 -> GAMMA/2(position)
  input/1 -> GAMMA/1(input)

== system GammaandTorqueMover/Disturbance added/Tube MPC plus D/MLPM Plant1/PINV ==
  input : Inport
  position : Inport  Port=2
  Constant1 : Constant  Value=-0.0715
  Constant10 : Constant  Value=3.9021
  Constant11 : Constant  Value=0.0508
  Constant2 : Constant  Value=3.14159265
  Constant3 : Constant  Value=-0.0203
  Constant4 : Constant  Value=-0.0146
  Constant5 : Constant  Value=-0.123
  Constant6 : Constant  Value=-0.1046
  Constant7 : Constant  Value=-87.14
  Constant8 : Constant  Value=5.5209
  Constant9 : Constant  Value=3.9021
  GAMMA : MATLAB Function  TreatAsAtomicUnit=on
  Scope : Scope
  Current : Outport
  wires:
  GAMMA/1(output) -> Scope/1, Current/1  "Gamma_PINV_output"
  input/1 -> GAMMA/1(input)
  position/1 -> GAMMA/2(position)
  Constant2/1 -> GAMMA/13(PI)
  Constant11/1 -> GAMMA/3(TAU)
  Constant7/1 -> GAMMA/4(BETA_K)
  Constant10/1 -> GAMMA/5(ALPHA_X)
  Constant9/1 -> GAMMA/6(ALPHA_Y)
  Constant8/1 -> GAMMA/7(ALPHA_Z)
  Constant1/1 -> GAMMA/8(ALPHA_M1)
  Constant6/1 -> GAMMA/9(ALPHA_M2)
  Constant5/1 -> GAMMA/10(BETA_M1)
  Constant3/1 -> GAMMA/11(BETA_M2)
  Constant4/1 -> GAMMA/12(ALPHA_RZ)

== system GammaandTorqueMover/Disturbance added/Tube MPC plus D/Subsystem/Gamma ==
  input : Inport
  position : Inport  Port=2
  Constant1 : Constant  Value=-0.0715
  Constant10 : Constant  Value=3.9021
  Constant11 : Constant  Value=0.0508
  Constant2 : Constant  Value=3.14159265
  Constant3 : Constant  Value=-0.0203
  Constant4 : Constant  Value=-0.0146
  Constant5 : Constant  Value=-0.123
  Constant6 : Constant  Value=-0.1046
  Constant7 : Constant  Value=-87.14
  Constant8 : Constant  Value=5.5209
  Constant9 : Constant  Value=3.9021
  GAMMA : MATLAB Function  TreatAsAtomicUnit=on
  Scope : Scope
  net_wrench : Outport
  wires:
  input/1 -> GAMMA/1(input)
  position/1 -> GAMMA/2(position)
  Constant2/1 -> GAMMA/13(PI)
  Constant11/1 -> GAMMA/3(TAU)
  Constant7/1 -> GAMMA/4(BETA_K)
  Constant10/1 -> GAMMA/5(ALPHA_X)
  Constant9/1 -> GAMMA/6(ALPHA_Y)
  Constant8/1 -> GAMMA/7(ALPHA_Z)
  Constant1/1 -> GAMMA/8(ALPHA_M1)
  Constant6/1 -> GAMMA/9(ALPHA_M2)
  Constant5/1 -> GAMMA/10(BETA_M1)
  Constant3/1 -> GAMMA/11(BETA_M2)
  Constant4/1 -> GAMMA/12(ALPHA_RZ)
  GAMMA/1(output) -> net_wrench/1, Scope/1  "Gamma_output"

== system GammaandTorqueMover/Disturbance added/Tube MPC plus D/Subsystem/PINV ==
  input : Inport
  position : Inport  Port=2
  Constant1 : Constant  Value=-0.0715
  Constant10 : Constant  Value=3.9021
  Constant11 : Constant  Value=0.0508
  Constant2 : Constant  Value=3.14159265
  Constant3 : Constant  Value=-0.0203
  Constant4 : Constant  Value=-0.0146
  Constant5 : Constant  Value=-0.123
  Constant6 : Constant  Value=-0.1046
  Constant7 : Constant  Value=-87.14
  Constant8 : Constant  Value=5.5209
  Constant9 : Constant  Value=3.9021
  GAMMA : MATLAB Function  TreatAsAtomicUnit=on
  Scope : Scope
  Current : Outport
  wires:
  Constant4/1 -> GAMMA/12(ALPHA_RZ)
  Constant3/1 -> GAMMA/11(BETA_M2)
  Constant5/1 -> GAMMA/10(BETA_M1)
  Constant6/1 -> GAMMA/9(ALPHA_M2)
  Constant1/1 -> GAMMA/8(ALPHA_M1)
  Constant8/1 -> GAMMA/7(ALPHA_Z)
  Constant9/1 -> GAMMA/6(ALPHA_Y)
  Constant10/1 -> GAMMA/5(ALPHA_X)
  Constant7/1 -> GAMMA/4(BETA_K)
  Constant11/1 -> GAMMA/3(TAU)
  Constant2/1 -> GAMMA/13(PI)
  position/1 -> GAMMA/2(position)
  input/1 -> GAMMA/1(input)
  GAMMA/1(output) -> Current/1, Scope/1  "Gamma_PINV_output"

== matlab function GammaandTorqueMover/PID/Subsystem/Gamma/GAMMA ==
  data: input input; position input; output output; TAU input; BETA_K input; ALPHA_X input; ALPHA_Y input; ALPHA_Z input; ALPHA_M1 input; ALPHA_M2 input; BETA_M1 input; BETA_M2 input; ALPHA_RZ input; PI input
function output = computeGammaBlock(input, position,TAU,BETA_K,ALPHA_X,ALPHA_Y,ALPHA_Z,ALPHA_M1,ALPHA_M2,BETA_M1,BETA_M2,ALPHA_RZ,PI)
% Call the generated function to compute Gamma
    X_M = position(1);
    Y_M = position(2);
    Z_M = position(3);
    ALPHA_ROTATION_M = position(4);
    BETA_ROTATION_M = position(5);
    GAMMA_ROTATION_M = position(6);
    Gamma = computeFullGammawithTorqueR4(X_M,Y_M,Z_M,ALPHA_ROTATION_M,BETA_ROTATION_M,GAMMA_ROTATION_M,TAU,BETA_K,ALPHA_X,ALPHA_Y,ALPHA_Z,ALPHA_M1,ALPHA_M2,BETA_M1,BETA_M2,ALPHA_RZ,PI);

    % Multiply Gamma by the input
    output = Gamma *input;
end

== matlab function GammaandTorqueMover/PID/Subsystem/MATLAB Function ==
  data: xdot output; u input; y output; x input
function [xdot, y] = System_SS_Model(u, x)
    % Parameters
    m = 6.6;            % Mass (kg)
    g = 9.81;           % Gravitational acceleration (m/s^2)
    
    % Moment of Inertia
    Ixx = 0.059;        % Moment of inertia around x-axis
    Iyy = 0.059;        % Moment of inertia around y-axis
    Izz = 0.12;         % Moment of inertia around z-axis
    
    % State vector x = [Px, Vx, Py, Vy, Pz, Vz, α, ω_x, β, ω_y, γ, ω_z]
    % Input vector u = [Fx, Fy, Fz, Tx, Ty, Tz]
    
    % State-Space Matrix (continuous time)
    A = zeros(12, 12);
    % Position-velocity couplings
    A(1,2) = 1;  % Px dot = Vx
    A(3,4) = 1;  % Py dot = Vy
    A(5,6) = 1;  % Pz dot = Vz
    A(7,8) = 1;  % α dot = ω_x
    A(9,10) = 1; % β dot = ω_y
    A(11,12) = 1;% γ dot = ω_z
    
    % Input Matrix (continuous time)
    B = zeros(12, 6);
    % Force to acceleration conversion
    B(2,1) = 1/m;    % Fx -> ax
    B(4,2) = 1/m;    % Fy -> ay
    B(6,3) = 1/m;    % Fz -> az
    % Torque to angular acceleration conversion
    B(8,4) = 1/Ixx;  % Tx -> α_ddot
    B(10,5) = 1/Iyy; % Ty -> β_ddot
    B(12,6) = 1/Izz; % Tz -> γ_ddot
    
    % Gravitational effect (constant acceleration in z direction)
    gravity = zeros(12,1);
    gravity(6) = -g;  % Acceleration in z direction
    
    % State derivative (continuous time)
    xdot = A * x + B * u + gravity;
    
    % Output equation: Only positions and orientations
    % Positions: Px (x(1)), Py (x(3)), Pz (x(5))
    % Orientations: α (x(7)), β (x(9)), γ (x(11))
    y = [ x(1); x(3); x(5); x(7); x(9); x(11) ];
end

== matlab function GammaandTorqueMover/Plant Verification/Gamma/GAMMA ==
  data: input input; position input; output output; TAU input; BETA_K input; ALPHA_X input; ALPHA_Y input; ALPHA_Z input; ALPHA_M1 input; ALPHA_M2 input; BETA_M1 input; BETA_M2 input; ALPHA_RZ input; PI input
function output = computeGammaBlock(input, position,TAU,BETA_K,ALPHA_X,ALPHA_Y,ALPHA_Z,ALPHA_M1,ALPHA_M2,BETA_M1,BETA_M2,ALPHA_RZ,PI)
% Call the generated function to compute Gamma
    X_M = position(1);
    Y_M = position(2);
    Z_M = position(3);
    ALPHA_ROTATION_M = position(4);
    BETA_ROTATION_M = position(5);
    GAMMA_ROTATION_M = position(6);
    Gamma = computeFullGammawithTorqueR4(X_M,Y_M,Z_M,ALPHA_ROTATION_M,BETA_ROTATION_M,GAMMA_ROTATION_M,TAU,BETA_K,ALPHA_X,ALPHA_Y,ALPHA_Z,ALPHA_M1,ALPHA_M2,BETA_M1,BETA_M2,ALPHA_RZ,PI);

    % Multiply Gamma by the input
    output = Gamma *input;
end
